simulink model "TestHarness"  (R2025b)
settings: Solver=VariableStepAuto  StartTime=0.0  StopTime=16  RelTol=1e-3  AbsTol=1e-3
PreLoadFcn:
  | SimulationTime = 10;
  | run('Harnessparm.m');
  | Choice=1;
undefined symbols (not defined in the file): base, Base, GFLBatteryController, loadl, pll, PVController, PVInverter, scan, Ts
libraries: nesl_utility x11, ee_lib x10, eeTransforms x7, fl_lib x5, eeSinusoidalMeasurementV2 x2, slpidlib x2, eeGeneralControl x2
settings Model: SimulationMode=accelerator  Creator=rajarshd  LastModifiedBy=rajarshd
settings SolverCC: AutoScaleAbsTol=off  AlgebraicLoopSolver=TrustRegion  MaxZcPerStep=1.0
settings DataIOCC: SaveOutput=off  DSMLogging=off  SaveTime=off  ReturnWorkspaceOutputsName=Data
settings DebuggingCC: UnconnectedInputMsg=warning  UnconnectedOutputMsg=warning  UnconnectedLineMsg=warning  SymbolicDimsDataTypeCodeGenerationDiagnostic=none
settings ModelReferenceCC: EnableRefExpFcnMdlSchedulingChecks=on
settings SFSimCC: CustomCodeUndefinedFunction=UseInterfaceOnly
settings RTWCC: GPUComputeCapability=3.5  DLArmComputeVersion=19.05
settings SimscapeCC: SimscapeLogType=all  SimscapeLogSimulationStatistics=on  SimscapeLogDataHistory=10000.0

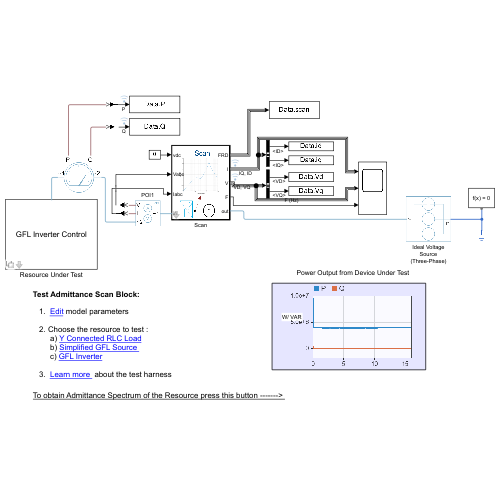
[thumbnail: Simulink's stored preview of the top-level diagram]
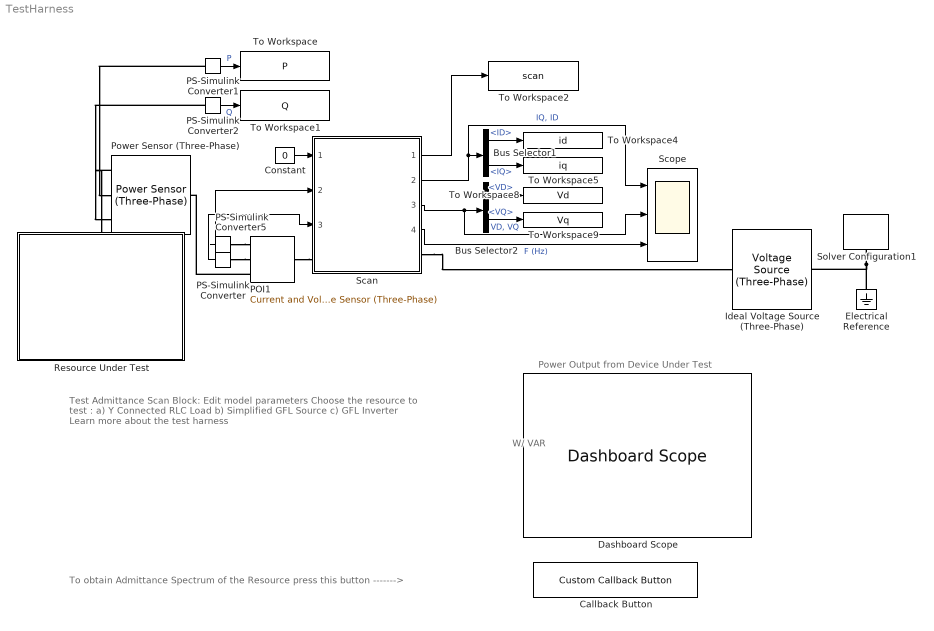
== system TestHarness ==
  note: W/ VAR
  note: Power Output from Device Under Test
  note: To obtain Admittance Spectrum of the Resource press this button ------->
  note: Test Admittance Scan Block:
      |
      | Edit model parameters
      |
      | Choose the resource to test :
      | a) Y Connected RLC Load
      | b) Simplified GFL Source
      | c) GFL Inverter
      |
      | Learn more about the test harness
  Bus Selector1 : BusSelector  OutputSignals=ID,IQ
  Bus Selector2 : BusSelector  OutputSignals=VD,VQ
  Callback Button : CustomCallbackButton  Configuration="{\"components\":[{\"name\":\"BackgroundImageComponent\",\"settings\":{\"image\":{\"size\":[0,0],\"src\":\"default\",\"srcOrientation\":\"Right\"},\"position\":[0,0,1,1]}},{\"name\":\"ButtonStateComponent\",\"settings\":{\"buttonType\":\"latch\",\"clickFcn\":\"Data=sim(bdroot);\\nmdl='TestHarness'; % Test model with IBR plant\\nadmittancescanPRBS(scan.Vd,scan.Vq,scan.Vdc,scan.f,Data.scan,modelorder,\\\"Y\\\") \",\"latched\":false,\"offValue\":null,\"onValue\":1,\"position\":[0,0,1,1],\"pressDelay\":\"500\",\"pressFcn\":\"\",\"repeatInterval\":\"0\",\"states\":[{\"horizontalAlignment\":\"center\",\"image\":{\"position\":[0,0,1,1],\"size\":[1,1],\"src\":\"default\",\"srcOrientation\":\"Right\"},\"label\":{\"color\":[1,1,1],\"icon\":{\"size\":[0,0],\"src\":\"default\",\"srcOrientation\":\"Right\"},\"iconOffset\":0,\"iconPlacement\":\"left\",\"opacity\":1,\"show\":true,\"text\":{\"content\":\"Admittance Scan\",\"font\":\"Helvetica\"}},\"labelOffset\":[0,0],\"verticalAlignment\":\"middle\"},{\"horizontalAlignment\":\"center\",\"image\":{\"position\":[0,0,1,1],\"size\":[1,1],\"src\":\"default\",\"srcOrientation\":\"Right\"},\"label\":{\"color\":[0.8509803921568627,0.3254901960784314,0.09803921568627451],\"icon\":{\"size\":[0,0],\"src\":\"default\",\"srcOrientation\":\"Right\"},\"iconOffset\":0,\"iconPlacement\":\"left\",\"opacity\":0,\"show\":true,\"text\":{\"content\":\"Admittance Scan\",\"font\":\"Helvetica\"}},\"labelOffset\":[-0.01428571428571429,-5.551115123125783e-17],\"verticalAlignment\":\"middle\"},{\"horizontalAlignment\":\"center\",\"image\":{\"position\":[0,0,1,1],\"size\":[1,1],\"src\":\"default\",\"srcOrientation\":\"Right\"},\"label\":{\"color\":[0.01176470588,0.01176470588,0.01176470588,1],\"icon\":{\"size\":[0,0],\"src\":\"default\",\"srcOrientation\":\"Right\"},\"iconOffset\":0,\"iconPlacement\":\"left\",\"opacity\":1,\"show\":true,\"text\":{\"content\":\"Admittance Scan\",\"font\":\"Helvetica\"}},\"labelOffset\":[0,0],\"verticalAlignment\":\"middle\"},{\"horizontalAlignment\":\"center\",\"image\":{\"position\":[0,0,1,1],\"size\":[1,1],\"src\":\"default\",\"srcOrientation\":\"Right\"},\"label\":{\"color\":[0.01176470588,0.01176470588,0.01176470588,1],\"icon\":{\"size\":[0,0],\"src\":\"default\",\"srcOrientation\":\"Right\"},\"iconOffset\":0,\"iconPlacement\":\"left\",\"opacity\":1,\"show\":true,\"text\":{\"content\":\"Admittance Scan\",\"font\":\"Helvetica\"}},\"labelOffset\":[0,0],\"verticalAlignment\":\"middle\"}]}},{\"name\":\"ForegroundImageComponent\",\"settings\":{\"image\":{\"size\":[0,0],\"src\":\"default\",\"srcOrientation\":\"Right\"},\"isForeground\":1,\"position\":[0,0,1,1]}}],\"derived\":{\"blockParameters\":{\"AutoActivate\":true,\"ButtonText\":\"Admittance Scan\",\"ButtonType\":\"Latch\",\"ClickFcn\":\"Data=sim(bdroot);\\nmdl='TestHarness'; % Test model with IBR plant\\nadmittancescanPRBS(scan.Vd,scan.Vq,scan.Vdc,scan.f,Data.scan,modelorder,\\\"Y\\\") \",\"OnValue\":1,\"PressDelay\":\"500\",\"PressFcn\":\"\",\"RepeatInterval\":\"0\",\"fixedAspectRatio\":\"off\"}},\"settings\":{\"BindingType\":\"standalone\",\"autoActivate\":true,\"backgroundColor\":[244,244,244,1],\"backgroundOffset\":0.2,\"backgroundOpacity\":1,\"fixedAspectRatio\":\"off\",\"foregroundColor\":[0.01176470588,0.01176470588,0.01176470588,1],\"migratedFromLegacy\":true,\"useBackgroundColor\":true,\"variant\":\"callback\",\"version\":\"R2025a\"},\"type\":\"Button\"}"  CustomBackgroundColor="{\"color\":[0,0.4470588235294118,0.7411764705882353],\"show\":true}"
  Constant : Constant  Value=0
  Dashboard Scope : DashboardScope  Ymin=0  Ymax=1e7  FontColor=[0.0, 0.0, 0.0]
  Electrical Reference : fl_lib/Electrical/Electrical Elements/Electrical Reference
  Ideal Voltage Source (Three-Phase) : ee_lib/Sources/Voltage Source (Three-Phase)  vline_rms=grid.voltage V  shift=0 deg  freq=grid.frequency Hz  impedance_option=0  SShortCircuit=1e6 A*V  XR=15  R=0.01 Ohm  L=0.2 mH  harmonic_option=0  harmonic_orders=[5, 7, 11, 13]  harmonic_ratios=[.1, .1, .1, .1]  G_parasitic=0 1/Ohm  I_specify=off  I_priority=None  I=[0, 0, 0] A  I_nominal_specify=off  I_nominal_value=1  I_nominal_unit=A
  POI1 : ee_lib/Sensors & Transducers/Current and Voltage Sensor (Three-Phase)  vMeasurementType=ee.enum.vmeasurement.lg  outputUnit=ee.enum.unit.si  SRated=base.mVA A*V  VRated=base.kV V  I_specify=off  I_priority=None  I=[0, 0, 0] A  I_nominal_specify=off  I_nominal_value=1  I_nominal_unit=A  V_specify=off  V_priority=None  V=[0, 0, 0] V  V_nominal_specify=off  V_nominal_value=1  V_nominal_unit=V
      settings: InternalSimscapePortConfiguration="{\"Bottom\":[],\"Left\":[{\"id\":\"N1\",\"label\":\"~1\",\"type\":\"foundation.electrical.three_phase\"}],\"Right\":[{\"id\":\"V_output\",\"label\":\"V\",\"type\":\"output\"},{\"id\":\"I_output\",\"label\":\"I\",\"type\":\"output\"},{\"id\":\"N2\",\"label\":\"~2\",\"type\":\"foundation.electrical.three_phase\"}],\"Top\":[]}"
  PS-Simulink Converter{,1..2,5} (4 alike) : nesl_utility/PS-Simulink Converter  PhysicalDomain=network_engine_domain  SubClassName=ps_output  LeftPortType=input  RightPortType=output  PseudoPeriodic=off  Frequencies=[]  VectorFormat=inherit  Unit=inherit  AffineConversion=off
  Power Sensor (Three-Phase) : ee_lib/Sensors & Transducers/Power Sensor (Three-Phase)  load_type=ee.enum.passive.type_balanced.balanced  f0=60 Hz
      settings: InternalSimscapePortConfiguration="{\"Bottom\":[],\"Left\":[{\"id\":\"N1\",\"label\":\"~1\",\"type\":\"foundation.electrical.three_phase\"}],\"Right\":[{\"id\":\"N2\",\"label\":\"~2\",\"type\":\"foundation.electrical.three_phase\"}],\"Top\":[{\"id\":\"Pm\",\"label\":\"P\",\"type\":\"output\"},{\"id\":\"Qm\",\"label\":\"Q\",\"type\":\"output\"}]}"
  Resource Under Test : Subsystem  Variant=on  VariantControl=Subsystem2  mask{Choice=GFL BESS}
      mask prompts: Choice "Choose Resource"
      mask TypeOptions Choice: Y Connected Load | Simplified GFL Source | GFL BESS
  Scan : Subsystem  ReferencedSubsystem=ScanBlockwithDC  F0=grid.frequency  Theta0=0  Kp_LF=pll.kp  Ki_LF=pll.ki  Ts=Ts  voltage=Base.KV_base_new  voltagedc=0  mva=base.mVA  Amplitude=scan.Vd  Amplitude1=scan.Vq  Amplitudedc=scan.Vdc  f=scan.f  T=1/scan.samplingfrequency  Tdis=scan.start  Tend=scan.end  VSelect=Equivalent Series Voltage (V)  Hold=No
  Scope : Scope  NumInputPorts=3
      settings: ActiveDisplayYMinimum=-3286.03322  ActiveDisplayYMaximum=550.92742
  Solver Configuration1 : nesl_utility/Solver Configuration  PhysicalDomain=network_engine_domain  SubClassName=solver  LeftPortType=input  RightPortType=generic  Tones=[]  Harmonics=[]  SimulateNoise=off  Profile=off  UseLocalSampling=off  EnableSwitchedLinearOptims=on  FrequencyDomain=off  UseCCode=off  RelTol=0.001  AbsTol=1e-06  MinStep=1e-09  ToWorkspace=off  RevertToSquareIcSolve=off  NumHomotopyIterations=100  PhasorMode=off  PhasorModeNumHarmonics=1  ConsistencySolver=NEWTON_XTOL_AFTER_FTOL  IndexReductionMethod=None  DoDC=off  ResidualTolerance=1e-3  ConsistencyTolSource=GLOBAL  ConsistencyAbsTol=0.001  ConsistencyRelTol=0.001  ConsistencyTolFactor=0.001  UseLocalSolver=on  LocalSolverChoice=NE_BACKWARD_EULER_ADVANCER  ResolveIndetEquations=off  FunctionEvalNumThread=1  LocalSolverSampleTime=5e-5  DoFixedCost=on  MaxNonlinIter=1  MaxModeIter=2  ComputeImpulses=off  ImpulseIterations=2  LinearAlgebra=Sparse  LinearAlgebraNumThread=0  EquationFormulation=NE_TIME_EF  DelaysMemoryBudget=1024  AutomaticFiltering=on  FilteringTimeConstant=0.001  PartitionStorageMethod=AS_NEEDED  PartitionMemoryBudget=1024  PartitionMethod=ROBUST  MultibodyUseLocalSolver=off  MultibodyLocalSolverChoice=ODE1  MultibodyLocalSolverSampleTime=0.001
  To Workspace : ToWorkspace  VariableName=P  SaveFormat=Timeseries  SampleTime=-1
  To Workspace1 : ToWorkspace  VariableName=Q  SaveFormat=Timeseries  SampleTime=-1
  To Workspace2 : ToWorkspace  VariableName=scan  SaveFormat=Timeseries  SampleTime=-1
  To Workspace4 : ToWorkspace  VariableName=id  SaveFormat=Timeseries  SampleTime=-1
  To Workspace5 : ToWorkspace  VariableName=iq  SaveFormat=Timeseries  SampleTime=-1
  To Workspace8 : ToWorkspace  VariableName=Vd  SaveFormat=Timeseries  SampleTime=-1
  To Workspace9 : ToWorkspace  VariableName=Vq  SaveFormat=Timeseries  SampleTime=-1
  wires:
  PS-Simulink Converter1/1 -> To Workspace/1  "P"
  PS-Simulink Converter2/1 -> To Workspace1/1  "Q"
  Scan/2 -> Scope/1, Bus Selector1/1  "IQ, ID"
  Scan/1 -> To Workspace2/1
  Scan/4 -> Scope/3  "F (Hz)"
  Scan/3 -> Scope/2, Bus Selector2/1  "VD, VQ"
  Bus Selector1/1 -> To Workspace4/1  "<ID>"
  Bus Selector1/2 -> To Workspace5/1  "<IQ>"
  Bus Selector2/1 -> To Workspace8/1  "<VD>"
  Bus Selector2/2 -> To Workspace9/1  "<VQ>"
  Constant/1 -> Scan/1
  PS-Simulink Converter5/1 -> Scan/2
  PS-Simulink Converter/1 -> Scan/3
  connections:
  PS-Simulink Converter1/LConn1 -- Power Sensor (Three-Phase)/LConn2
  PS-Simulink Converter2/LConn1 -- Power Sensor (Three-Phase)/LConn3
  Scan/RConn1 -- Ideal Voltage Source (Three-Phase)/RConn1
  Solver Configuration1/RConn1 -- Ideal Voltage Source (Three-Phase)/LConn1 -- Electrical Reference/LConn1
  PS-Simulink Converter/LConn1 -- POI1/RConn2
  PS-Simulink Converter5/LConn1 -- POI1/RConn1
  Power Sensor (Three-Phase)/LConn1 -- Resource Under Test/LConn1
  POI1/LConn1 -- Scan/LConn1
  POI1/RConn3 -- Power Sensor (Three-Phase)/RConn1

== system TestHarness/Resource Under Test ==
  " GFL Source" : Subsystem  VariantControl=Choice==2  mask{axis=D Axis, Denominator=[1 2*0.1*(2*pi*40) (2*pi*40)^2], Numerator=1e3, Numerator1=1e3, Denominator1=[1 +2*0.1*(2*pi*40) (2*pi*40)^2]}
      mask prompts: axis "TF Along:"; Denominator "D axis TF Denominator"; Numerator "D axis TF Numerator"; Numerator1 "Q axis TF Numerator"; Denominator1 "Q axis TF Denominator"
      mask TypeOptions axis: D Axis | Q Axis
      mask Display:
      | g=get_param(gcb,'axis');
      | if(g=='D Axis')
      | den = get_param(gcb, 'Denominator');
      | nu  = get_param(gcb, 'Numerator');
      | disp('Admittance TF along D axis:\n\n\n\n\n');
      | den1 = get_param(gcb, 'Denominator1');
      | nu1  = get_param(gcb, 'Numerator1');
      | dpoly(nu, den,'s');
      | end
      | if(g=='Q Axis')
      | den1 = get_param(gcb, 'Denominator1');
      | nu1  = get_param(gcb, 'Numerator1');
      | disp('Admittance TF along Q axis:\n\n\n\n\n');
      | den1 = get_param(gcb, 'Denominator1');
      | nu1  = get_param(gcb, 'Numerator1');
      | dpoly(nu1, den1,'s');
      | end
  GFL : Subsystem  VariantControl=Choice==3
      mask Display: disp('GFL Inverter Control');
  Wye-Connected Load : Subsystem  VariantControl=Choice==1  mask{C=loadl.c, L=loadl.l, R=loadl.r}
      mask prompts: C "physmod:ee:library:comments:passive:rlc_assemblies:wye:Xabc:C"; L "physmod:ee:library:comments:passive:rlc_assemblies:wye:Xabc:L"; R "physmod:ee:library:comments:passive:rlc_assemblies:wye:Xabc:R"
      mask TypeOptions C: Wye-Connected Load/C
      mask TypeOptions L: Wye-Connected Load/L
      mask TypeOptions R: Wye-Connected Load/R
      mask Display: disp('Y Connected \n R L C series Load');
  Conn1 : PMIOPort  Side=Left

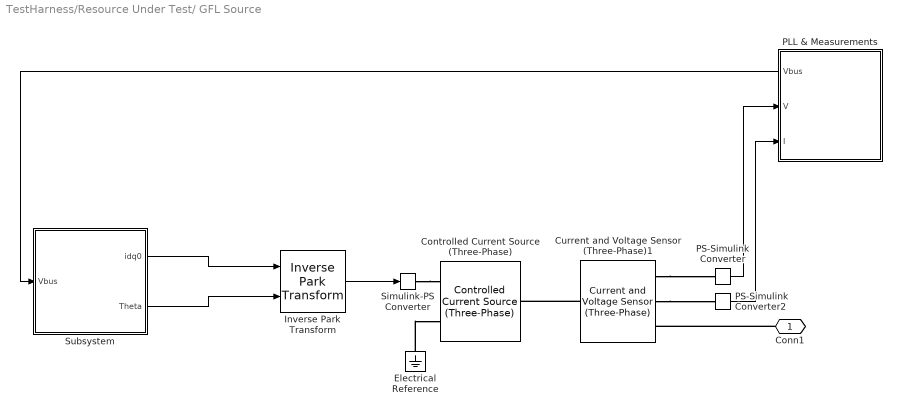
== system TestHarness/Resource Under Test/ GFL Source ==
  Controlled Current Source (Three-Phase) : ee_lib/Sources/Controlled Current Source (Three-Phase)  input_option=ee.enum.inputType.instantaneous  FRated=60 Hz
      settings: InternalSimscapePortConfiguration="{\"Bottom\":[],\"Left\":[{\"id\":\"S\",\"label\":\"S\",\"type\":\"input\"},{\"id\":\"n\",\"label\":\"n\",\"type\":\"foundation.electrical.electrical\"}],\"Right\":[{\"id\":\"N\",\"label\":\"~\",\"type\":\"foundation.electrical.three_phase\"}],\"Top\":[]}"
  Current and Voltage Sensor (Three-Phase)1 : ee_lib/Sensors & Transducers/Current and Voltage Sensor (Three-Phase)  vMeasurementType=ee.enum.vmeasurement.lg  outputUnit=ee.enum.unit.si  SRated=base.mVA A*V  VRated=base.kV V  I_specify=off  I_priority=None  I=[0, 0, 0] A  I_nominal_specify=off  I_nominal_value=1  I_nominal_unit=A  V_specify=off  V_priority=None  V=[0, 0, 0] V  V_nominal_specify=off  V_nominal_value=1  V_nominal_unit=V
      settings: InternalSimscapePortConfiguration="{\"Bottom\":[],\"Left\":[{\"id\":\"N1\",\"label\":\"~1\",\"type\":\"foundation.electrical.three_phase\"}],\"Right\":[{\"id\":\"V_output\",\"label\":\"V\",\"type\":\"output\"},{\"id\":\"I_output\",\"label\":\"I\",\"type\":\"output\"},{\"id\":\"N2\",\"label\":\"~2\",\"type\":\"foundation.electrical.three_phase\"}],\"Top\":[]}"
  Electrical Reference : fl_lib/Electrical/Electrical Elements/Electrical Reference
  Inverse Park Transform : eeTransforms/Inverse Park Transform  AxisAlignment=Q-axis  PowerInvariant=on
      settings: LibrarySourceBlock=|
      | ee_sl_lib/Mathematical
      | Transforms/Inverse
      | Park Transform
  PLL & Measurements : Subsystem
      settings: PortSchema="{\"entries\":[{\"content\":{\"sides\":[{\"content\":{\"connectorIds\":[\"Out1\",\"In1\",\"In2\"]},\"type\":\"ConnectorPlacement.EquallySpacedRectSide\",\"uuid\":\"76485780-20fe-4fcf-8224-69648da6ed2a\"},{\"content\":{\"connectorIds\":[],\"side\":\"RIGHT\"},\"type\":\"ConnectorPlacement.EquallySpacedRectSide\",\"uuid\":\"f19a6390-e634-42c7-8d46-4cd80cbab182\"},{\"content\":{\"connectorIds\":[],\"side\":\"TOP\"},\"type\":\"ConnectorPlacement.EquallySpacedRectSide\",\"uuid\":\"87682f72-1844-428e-be70-ad7ca3191ee3\"}]},\"type\":\"ConnectorPlacement.EquallySpacedConnector\",\"uuid\":\"f2136b07-48ec-402b-adb3-18c0bac2157c\"}],\"packageUris\":[\"http://schema.mathworks.com/mf0/Connector/R2020b\"],\"version\":\"1.0\"}"
      mask Display: image('$imagefile'); % Use "Edit Image" on toolstrip to change.
  PS-Simulink Converter : nesl_utility/PS-Simulink Converter  PhysicalDomain=network_engine_domain  SubClassName=ps_output  LeftPortType=input  RightPortType=output  PseudoPeriodic=off  Frequencies=[]  VectorFormat=inherit  Unit=inherit  AffineConversion=off
  PS-Simulink Converter2 : nesl_utility/PS-Simulink Converter  PhysicalDomain=network_engine_domain  SubClassName=ps_output  LeftPortType=input  RightPortType=output  PseudoPeriodic=off  Frequencies=[]  VectorFormat=inherit  Unit=inherit  AffineConversion=off
  Simulink-PS Converter : nesl_utility/Simulink-PS Converter  PhysicalDomain=network_engine_domain  SubClassName=ps_input  LeftPortType=input  RightPortType=output  PseudoPeriodic=off  Frequencies=[]  NoiseDistribution=none  NoiseParameters=[]  Unit=1  AffineConversion=off  FilteringAndDerivatives=provide  SimscapeFilterOrder=1  InputFilterTimeConstant=0.001  UdotUserProvided=0
  Subsystem : Subsystem
  Conn1 : PMIOPort  Side=Left
  wires:
  PS-Simulink Converter/1 -> PLL & Measurements/1(V)
  PS-Simulink Converter2/1 -> PLL & Measurements/2(I)
  PLL & Measurements/1(Vbus) -> Subsystem/1(Vbus)
  Subsystem/1(idq0) -> Inverse Park Transform/1
  Inverse Park Transform/1 -> Simulink-PS Converter/1
  Subsystem/2(Theta) -> Inverse Park Transform/2
  connections:
  Current and Voltage Sensor (Three-Phase)1/RConn2 -- PS-Simulink Converter2/LConn1
  Current and Voltage Sensor (Three-Phase)1/RConn1 -- PS-Simulink Converter/LConn1
  Simulink-PS Converter/RConn1 -- Controlled Current Source (Three-Phase)/LConn1
  Electrical Reference/LConn1 -- Controlled Current Source (Three-Phase)/LConn2
  Conn1/RConn1 -- Current and Voltage Sensor (Three-Phase)1/RConn3
  Current and Voltage Sensor (Three-Phase)1/LConn1 -- Controlled Current Source (Three-Phase)/RConn1

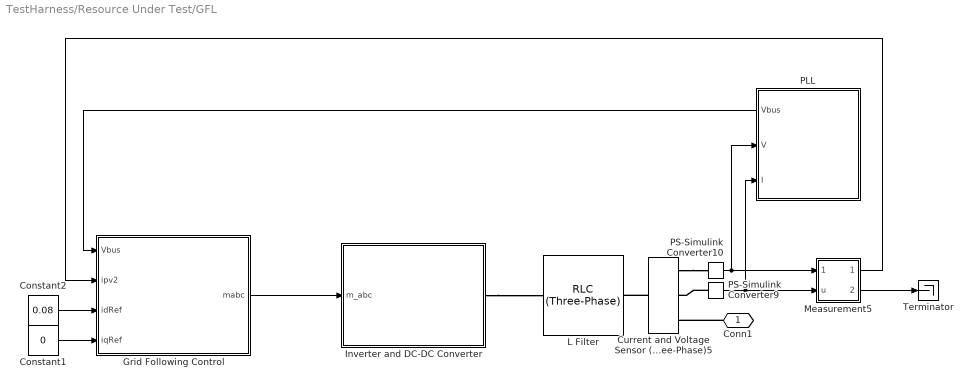
== system TestHarness/Resource Under Test/GFL ==
  Constant1 : Constant  Value=0  SampleTime=Ts
  Constant2 : Constant  Value=0.08  SampleTime=Ts
  Current and Voltage Sensor (Three-Phase)5 : ee_lib/Sensors & Transducers/Current and Voltage Sensor (Three-Phase)  vMeasurementType=ee.enum.vmeasurement.lg  outputUnit=ee.enum.unit.pu  SRated=Base.MVA_base_new A*V  VRated=Base.KV_base_new V  I_specify=off  I_priority=None  I=[0, 0, 0] A  I_nominal_specify=off  I_nominal_value=1  I_nominal_unit=A  V_specify=off  V_priority=None  V=[0, 0, 0] V  V_nominal_specify=off  V_nominal_value=1  V_nominal_unit=V
      settings: InternalSimscapePortConfiguration="{\"Bottom\":[],\"Left\":[{\"id\":\"N1\",\"label\":\"~1\",\"type\":\"foundation.electrical.three_phase\"}],\"Right\":[{\"id\":\"V_output\",\"label\":\"V\",\"type\":\"output\"},{\"id\":\"I_output\",\"label\":\"I\",\"type\":\"output\"},{\"id\":\"N2\",\"label\":\"~2\",\"type\":\"foundation.electrical.three_phase\"}],\"Top\":[]}"
  Grid Following Control : Subsystem  VariantControl=BESSGridSupporting
      mask Display: image('$imagefile'); % Use "Edit Image" on toolstrip to change.
  Inverter and DC-DC Converter : Subsystem
  L Filter : ee_lib/Passive/RLC Assemblies/RLC (Three-Phase)  port_option=ee.enum.threePhasePort.composite  component_structure=ee.enum.rlc.structure.L  R=1e-3 Ohm  L=PVInverter.L*10 H  C=1e-6 F  R_parasitic=0 Ohm  G_parasitic=0 1/Ohm  IL_specify=off  IL_priority=High  IL=[0, 0, 0] A  IL_nominal_specify=off  IL_nominal_value=1  IL_nominal_unit=A  VC_specify=off  VC_priority=High  VC=[0, 0, 0] V  VC_nominal_specify=off  VC_nominal_value=1  VC_nominal_unit=V
      settings: InternalSimscapePortConfiguration="{\"Bottom\":[],\"Left\":[{\"id\":\"N1\",\"label\":\"~1\",\"type\":\"foundation.electrical.three_phase\"}],\"Right\":[{\"id\":\"N2\",\"label\":\"~2\",\"type\":\"foundation.electrical.three_phase\"}],\"Top\":[]}"
  Measurement5 : Subsystem
  "PLL " : Subsystem
      settings: PortSchema="{\"entries\":[{\"content\":{\"sides\":[{\"content\":{\"connectorIds\":[\"Out1\",\"In1\",\"In2\"]},\"type\":\"ConnectorPlacement.EquallySpacedRectSide\",\"uuid\":\"76485780-20fe-4fcf-8224-69648da6ed2a\"},{\"content\":{\"connectorIds\":[],\"side\":\"RIGHT\"},\"type\":\"ConnectorPlacement.EquallySpacedRectSide\",\"uuid\":\"f19a6390-e634-42c7-8d46-4cd80cbab182\"},{\"content\":{\"connectorIds\":[],\"side\":\"TOP\"},\"type\":\"ConnectorPlacement.EquallySpacedRectSide\",\"uuid\":\"87682f72-1844-428e-be70-ad7ca3191ee3\"}]},\"type\":\"ConnectorPlacement.EquallySpacedConnector\",\"uuid\":\"f2136b07-48ec-402b-adb3-18c0bac2157c\"}],\"packageUris\":[\"http://schema.mathworks.com/mf0/Connector/R2020b\"],\"version\":\"1.0\"}"
      mask Display: image('$imagefile'); % Use "Edit Image" on toolstrip to change.
  PS-Simulink Converter10 : nesl_utility/PS-Simulink Converter  PhysicalDomain=network_engine_domain  SubClassName=ps_output  LeftPortType=input  RightPortType=output  PseudoPeriodic=off  Frequencies=[]  VectorFormat=inherit  Unit=inherit  AffineConversion=off
  PS-Simulink Converter9 : nesl_utility/PS-Simulink Converter  PhysicalDomain=network_engine_domain  SubClassName=ps_output  LeftPortType=input  RightPortType=output  PseudoPeriodic=off  Frequencies=[]  VectorFormat=inherit  Unit=inherit  AffineConversion=off
  Terminator : Terminator
  Conn1 : PMIOPort  Side=Left
  wires:
  Grid Following Control/1(mabc) -> Inverter and DC-DC Converter/1(m_abc)
  PS-Simulink Converter9/1 -> "PLL "/2(I), Measurement5/2(u)
  PS-Simulink Converter10/1 -> "PLL "/1(V), Measurement5/1(In1)
  Measurement5/2(Bat) -> Terminator/1
  Measurement5/1(ipv1) -> Grid Following Control/2(ipv2)
  "PLL "/1(Vbus) -> Grid Following Control/1(Vbus)
  Constant2/1 -> Grid Following Control/3(idRef)
  Constant1/1 -> Grid Following Control/4(iqRef)
  connections:
  Conn1/RConn1 -- Current and Voltage Sensor (Three-Phase)5/RConn3
  Inverter and DC-DC Converter/RConn1 -- L Filter/LConn1
  Current and Voltage Sensor (Three-Phase)5/LConn1 -- L Filter/RConn1
  Current and Voltage Sensor (Three-Phase)5/RConn1 -- PS-Simulink Converter10/LConn1
  PS-Simulink Converter9/LConn1 -- Current and Voltage Sensor (Three-Phase)5/RConn2

== system TestHarness/Resource Under Test/Wye-Connected Load ==
  Electrical Reference : fl_lib/Electrical/Electrical Elements/Electrical Reference
  Wye-Connected Load : ee_lib/Passive/RLC Assemblies/Wye-Connected Load  port_option=ee.enum.threePhasePort.composite  parameterization=ee.enum.rlc.parameterization.direct  component_structure=ee.enum.rlc.structure.SeriesRLC  component_structure_PQ=ee.enum.rlc.structure.SeriesRL  R=R Ohm  L=L H  C=C F  VRated=24e3 V  FRated=60 Hz  P=1e3 W  Qpos=1e2 A*V  Qneg=-1e2 A*V  R_parasitic=0 Ohm  G_parasitic=0 1/Ohm  R_parasitic_PQ=0 Ohm  G_parasitic_PQ=0 1/Ohm  Vmag0=24e3 V  Vang0=0 deg  Freq0=60 Hz  IL_specify=off  IL_priority=High  IL=[0, 0, 0] A  IL_nominal_specify=off  IL_nominal_value=1  IL_nominal_unit=A  VC_specify=off  VC_priority=High  VC=[0, 0, 0] V  VC_nominal_specify=off  VC_nominal_value=1  VC_nominal_unit=V
  Conn1 : PMIOPort  Side=Left
  connections:
  Conn1/RConn1 -- Wye-Connected Load/LConn1
  Electrical Reference/LConn1 -- Wye-Connected Load/RConn1

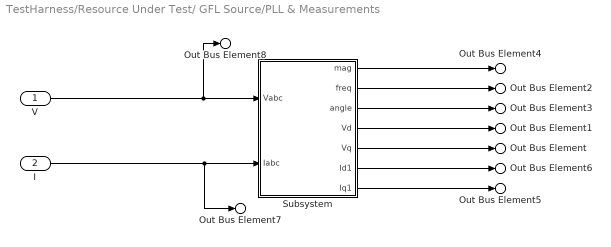
== system TestHarness/Resource Under Test/ GFL Source/PLL & Measurements ==
  V : Inport
  I : Inport  Port=2
  Subsystem : Subsystem
  Out Bus Element : Outport  PortName=Vbus  Element=Vq
  Out Bus Element1 : Outport  PortName=Vbus  Element=Vd
  Out Bus Element2 : Outport  PortName=Vbus  Element=w
  Out Bus Element3 : Outport  PortName=Vbus  Element=Theta
  Out Bus Element4 : Outport  PortName=Vbus  Element=Vmag
  Out Bus Element5 : Outport  PortName=Vbus  Element=Iq
  Out Bus Element6 : Outport  PortName=Vbus  Element=Id
  Out Bus Element7 : Outport  PortName=Vbus  Element=Iabc
  Out Bus Element8 : Outport  PortName=Vbus  Element=Vabc
  wires:
  Subsystem/2(freq) -> Out Bus Element2/1
  Subsystem/5(Vq) -> Out Bus Element/1
  Subsystem/3(angle) -> Out Bus Element3/1
  Subsystem/4(Vd) -> Out Bus Element1/1
  V/1 -> Out Bus Element8/1, Subsystem/1(Vabc)
  Subsystem/1(mag) -> Out Bus Element4/1
  I/1 -> Out Bus Element7/1, Subsystem/2(Iabc)
  Subsystem/7(Iq1) -> Out Bus Element5/1
  Subsystem/6(Id1) -> Out Bus Element6/1

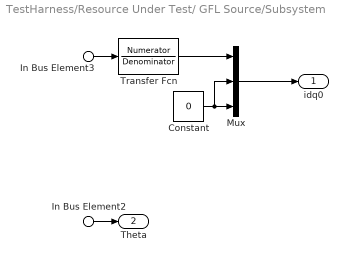
== system TestHarness/Resource Under Test/ GFL Source/Subsystem ==
  In Bus Element3 : Inport  PortName=Vbus  Element=Vd
  In Bus Element2 : Inport  PortName=Vbus  Element=Theta
  Constant : Constant  Value=0
  Mux : Mux  Inputs=3
  Transfer Fcn : TransferFcn  Numerator=Numerator  Denominator=Denominator
  idq0 : Outport
  Theta : Outport  Port=2
  wires:
  Mux/1 -> idq0/1
  In Bus Element2/1 -> Theta/1
  In Bus Element3/1 -> Transfer Fcn/1
  Constant/1 -> Mux/2, Mux/3
  Transfer Fcn/1 -> Mux/1

== system TestHarness/Resource Under Test/GFL/Grid Following Control ==
  In Bus Element : Inport  PortName=Vbus
  In Bus Element1 : Inport  Port=2  PortName=ipv2
  idRef : Inport  Port=3
  iqRef : Inport  Port=4
  GFL Battery Controller : Subsystem  mask{Vref=GFLBatteryController.V_ref, fref=GFLBatteryController.f_ref, Pref=GFLBatteryController.P_ref, Qref=GFLBatteryController.Q_ref, mp=GFLBatteryController.m_p, mv=GFLBatteryController.m_v, P=Real power, MVA=Base.MVA_base_new, zbase=Base.z_base, L=PVInverter.L*10, Imax=PVInverter.I_max_pu, Td=GFLBatteryController.Td, Kpic=PVController.Kp_ic, Kiic=PVController.Ki_ic, Kd=PVController.Kd}
      mask prompts: Vref "Voltage reference (PU)"; fref "Frequency reference (Hz)"; Pref "Real power reference (PU)"; Qref "Reactive power reference (PU)"; mp "Real power droop cofficient"; mv "Reactive power droop cofficient"; P "Priority mode"; MVA "Base Power (V*A)"; zbase "Base Impedance (Ohm)"; L "Filter Inductance (H)"; Imax "Inverter current limit (pu)"; Td "Sensor time delay (s)"; Kpic "Proportional gain"; Kiic "Integral gain"; Kd "Derevative gain"
      mask TypeOptions P: Real power  | Reactive power
      mask DialogControl Container4 Prompt: General
      mask DialogControl Container5 Prompt: Current Controller
      mask Display: image('$imagefile'); % Use "Edit Image" on toolstrip to change.
  mabc : Outport
  wires:
  In Bus Element/1 -> GFL Battery Controller/1(Vbus)
  In Bus Element1/1 -> GFL Battery Controller/2(ipv2)
  GFL Battery Controller/1(m_abc) -> mabc/1
  idRef/1 -> GFL Battery Controller/3(IdRef)
  iqRef/1 -> GFL Battery Controller/4(IqRef)

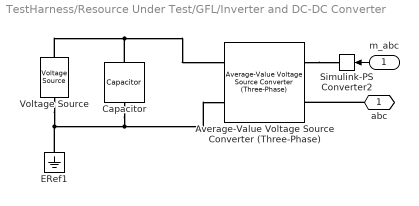
== system TestHarness/Resource Under Test/GFL/Inverter and DC-DC Converter ==
  m_abc : Inport
  Average-Value Voltage Source Converter (Three-Phase) : ee_lib/Semiconductors & Converters/Converters/Average-Value Voltage Source Converter (Three-Phase)  port_option=ee.enum.threePhasePort.composite  frequency_option=ee.enum.converters.frequency.variable  input_option=ee.enum.converters.inputOption.ModWave  FRated=60 Hz  losses_parameterization=ee.enum.converters.losses.fixed  Pfixed=1 W  ks=0.01  kc1=1.7 V  kc2=0.01 Ohm  Ploss_vect=[100, 800, 1870, 3250, 4900] W  Irms_vect=[10, 100, 200, 300, 400] A  Vdc_nom=300 V  thermal_mass=30000 J/K  temperature_specify=off  temperature_priority=High  temperature=298.15 K  temperature_nominal_specify=off  temperature_nominal_value=1  temperature_nominal_unit=K
      settings: InternalSimscapePortConfiguration="{\"Bottom\":[],\"Left\":[{\"id\":\"ModWave\",\"label\":\"ModWave\",\"type\":\"input\"},{\"id\":\"N\",\"label\":\"~\",\"type\":\"foundation.electrical.three_phase\"}],\"Right\":[{\"id\":\"p\",\"label\":\"+\",\"type\":\"foundation.electrical.electrical\"},{\"id\":\"n\",\"label\":\"-\",\"type\":\"foundation.electrical.electrical\"}],\"Top\":[]}"
  Capacitor : fl_lib/Electrical/Electrical Elements/Capacitor  c=GFMBatteryController.C_dc F  r=1e-6 Ohm  g=0 1/Ohm  i_specify=off  i_priority=None  i=0 A  i_nominal_specify=off  i_nominal_value=1  i_nominal_unit=A  v_specify=off  v_priority=None  v=6560*.5 V  v_nominal_specify=off  v_nominal_value=1  v_nominal_unit=V  vc_specify=on  vc_priority=None  vc=PVInverter.Vdc V  vc_nominal_specify=off  vc_nominal_value=1  vc_nominal_unit=V
  ERef1 : fl_lib/Electrical/Electrical Elements/Electrical Reference
  Simulink-PS Converter2 : nesl_utility/Simulink-PS Converter  PhysicalDomain=network_engine_domain  SubClassName=ps_input  LeftPortType=input  RightPortType=output  PseudoPeriodic=off  Frequencies=[]  NoiseDistribution=none  NoiseParameters=[]  Unit=1  AffineConversion=off  FilteringAndDerivatives=provide  SimscapeFilterOrder=1  InputFilterTimeConstant=0.001  UdotUserProvided=0
  Voltage Source : ee_lib/Sources/Voltage Source  dc_voltage=PVInverter.Vdc V  ac_voltage=0 V  ac_shift=0 rad  ac_frequency=60 Hz  noise_mode=ee.enum.sources.noise.Disabled  PSD=0 V^2/Hz  sample_time=1e-3 s  repeatability=ee.enum.sources.repeatability.NotRepeatable  user_seed=0  auto_seed=1872246315  i_specify=off  i_priority=None  i=0 A  i_nominal_specify=off  i_nominal_value=1  i_nominal_unit=A  v_specify=off  v_priority=None  v=0 V  v_nominal_specify=off  v_nominal_value=1  v_nominal_unit=V
  abc : PMIOPort  Side=Right
  wires:
  m_abc/1 -> Simulink-PS Converter2/1
  connections:
  Voltage Source/RConn1 -- ERef1/LConn1 -- Capacitor/RConn1 -- Average-Value Voltage Source Converter (Three-Phase)/RConn2
  Capacitor/LConn1 -- Voltage Source/LConn1 -- Average-Value Voltage Source Converter (Three-Phase)/RConn1
  Average-Value Voltage Source Converter (Three-Phase)/LConn1 -- Simulink-PS Converter2/RConn1
  abc/RConn1 -- Average-Value Voltage Source Converter (Three-Phase)/LConn2

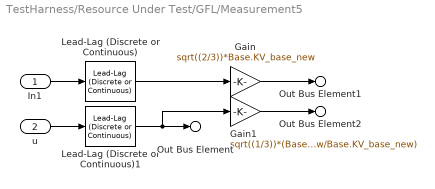
== system TestHarness/Resource Under Test/GFL/Measurement5 ==
  In1 : Inport
  u : Inport  Port=2
  Gain : Gain  Gain=sqrt((2/3))*Base.KV_base_new
  Gain1 : Gain  Gain=sqrt((1/3))*(Base.MVA_base_new/Base.KV_base_new)
  Lead-Lag (Discrete or Continuous) : eeGeneralControl/Lead-Lag (Discrete or Continuous)  T1=0  T2=PVController.t_sensor  B=inf  A=-inf  init_option=Inherited from block input  x0=0  Ts=Ts
      settings: LibrarySourceBlock=|
      | ee_sl_lib/General Control/Lead-Lag
      | (Discrete or Continuous)
  Lead-Lag (Discrete or Continuous)1 : eeGeneralControl/Lead-Lag (Discrete or Continuous)  T1=0  T2=PVController.t_sensor  B=inf  A=-inf  init_option=Inherited from block input  x0=0  Ts=Ts
      settings: LibrarySourceBlock=|
      | ee_sl_lib/General Control/Lead-Lag
      | (Discrete or Continuous)
  Out Bus Element : Outport  PortName=ipv1  Element=1
  Out Bus Element1 : Outport  Port=2  PortName=Bat  Element=Vabc_bat
  Out Bus Element2 : Outport  Port=2  PortName=Bat  Element=Iabc_bat
  wires:
  u/1 -> Lead-Lag (Discrete or Continuous)1/1
  Lead-Lag (Discrete or Continuous)1/1 -> Gain1/1, Out Bus Element/1
  In1/1 -> Lead-Lag (Discrete or Continuous)/1
  Lead-Lag (Discrete or Continuous)/1 -> Gain/1
  Gain/1 -> Out Bus Element1/1
  Gain1/1 -> Out Bus Element2/1

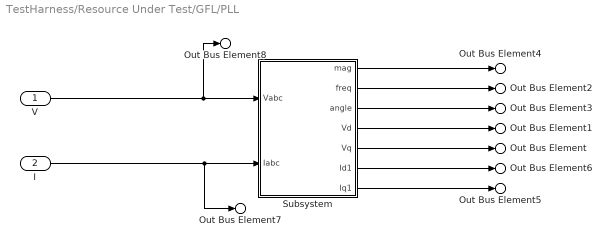
== system TestHarness/Resource Under Test/GFL/PLL  ==
  V : Inport
  I : Inport  Port=2
  Subsystem : Subsystem
  Out Bus Element : Outport  PortName=Vbus  Element=Vq
  Out Bus Element1 : Outport  PortName=Vbus  Element=Vd
  Out Bus Element2 : Outport  PortName=Vbus  Element=w
  Out Bus Element3 : Outport  PortName=Vbus  Element=Theta
  Out Bus Element4 : Outport  PortName=Vbus  Element=Vmag
  Out Bus Element5 : Outport  PortName=Vbus  Element=Iq
  Out Bus Element6 : Outport  PortName=Vbus  Element=Id
  Out Bus Element7 : Outport  PortName=Vbus  Element=Iabc
  Out Bus Element8 : Outport  PortName=Vbus  Element=Vabc
  wires:
  Subsystem/2(freq) -> Out Bus Element2/1
  Subsystem/5(Vq) -> Out Bus Element/1
  Subsystem/3(angle) -> Out Bus Element3/1
  Subsystem/4(Vd) -> Out Bus Element1/1
  V/1 -> Out Bus Element8/1, Subsystem/1(Vabc)
  Subsystem/1(mag) -> Out Bus Element4/1
  I/1 -> Out Bus Element7/1, Subsystem/2(Iabc)
  Subsystem/7(Iq1) -> Out Bus Element5/1
  Subsystem/6(Id1) -> Out Bus Element6/1

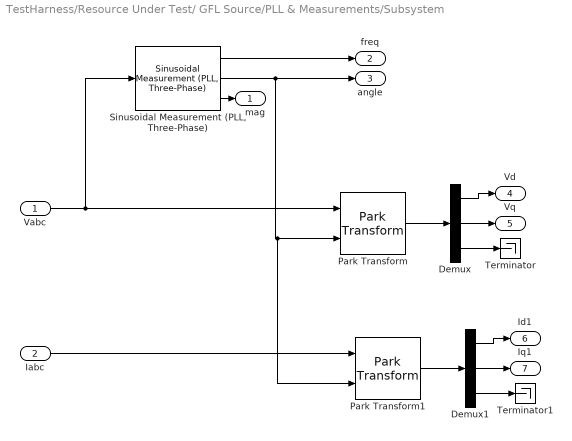
== system TestHarness/Resource Under Test/ GFL Source/PLL & Measurements/Subsystem ==
  Vabc : Inport
  Iabc : Inport  Port=2
  Demux : Demux  Outputs=3
  Demux1 : Demux  Outputs=3
  Park Transform : eeTransforms/Park Transform  AxisAlignment=Q-axis  PowerInvariant=on
  Park Transform1 : eeTransforms/Park Transform  AxisAlignment=Q-axis  PowerInvariant=on
  "Sinusoidal Measurement (PLL, Three-Phase)" : eeSinusoidalMeasurementV2/Sinusoidal Measurement (PLL, Three-Phase)  InputFilter=on  InputNormalization=off  Kp_LF=pll.kp/base.kV  Ki_LF=pll.ki /base.kV  F0=grid.frequency  Theta0=0  Ts=Ts
  Terminator : Terminator
  Terminator1 : Terminator
  mag : Outport
  freq : Outport  Port=2
  angle : Outport  Port=3
  Vd : Outport  Port=4
  Vq : Outport  Port=5
  Id1 : Outport  Port=6
  Iq1 : Outport  Port=7
  wires:
  Demux/3 -> Terminator/1
  Park Transform/1 -> Demux/1
  Demux/1 -> Vd/1
  Demux/2 -> Vq/1
  "Sinusoidal Measurement (PLL, Three-Phase)"/2 -> angle/1, Park Transform1/2, Park Transform/2
  "Sinusoidal Measurement (PLL, Three-Phase)"/1 -> freq/1
  "Sinusoidal Measurement (PLL, Three-Phase)"/3 -> mag/1
  Park Transform1/1 -> Demux1/1
  Demux1/1 -> Id1/1
  Demux1/2 -> Iq1/1
  Demux1/3 -> Terminator1/1
  Iabc/1 -> Park Transform1/1
  Vabc/1 -> "Sinusoidal Measurement (PLL, Three-Phase)"/1, Park Transform/1

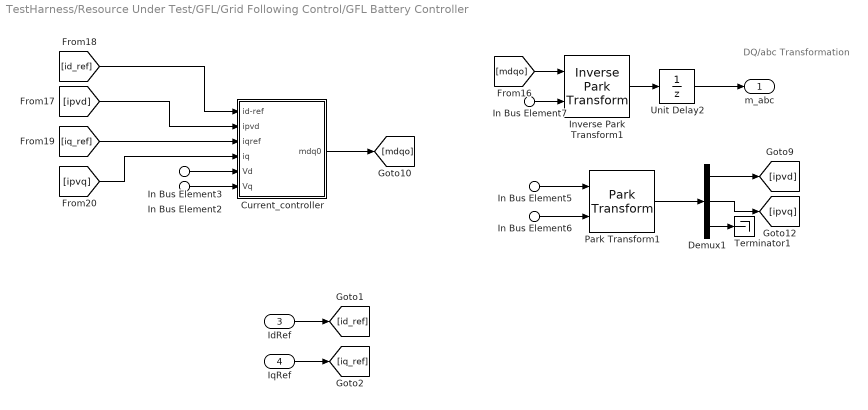
== system TestHarness/Resource Under Test/GFL/Grid Following Control/GFL Battery Controller ==
  note: DQ/abc Transformation
  In Bus Element3 : Inport  PortName=Vbus  Element=Vd
  In Bus Element2 : Inport  PortName=Vbus  Element=Vq
  In Bus Element6 : Inport  PortName=Vbus  Element=Theta
  In Bus Element7 : Inport  PortName=Vbus  Element=Theta
  In Bus Element5 : Inport  Port=2  PortName=ipv2  Element=1
  IdRef : Inport  Port=3
  IqRef : Inport  Port=4
  Current_controller : Subsystem
  Demux1 : Demux  Outputs=3
  Inverse Park Transform1 : eeTransforms/Inverse Park Transform  AxisAlignment=Q-axis  PowerInvariant=off
  Park Transform1 : eeTransforms/Park Transform  AxisAlignment=Q-axis  PowerInvariant=off
  Terminator1 : Terminator
  Unit Delay2 : UnitDelay  SampleTime=Ts  HasFrameUpgradeWarning=on
  m_abc : Outport
  wires:
  In Bus Element2/1 -> Current_controller/6(Vq)
  Current_controller/1(mdq0) -> [mdqo]
  Inverse Park Transform1/1 -> Unit Delay2/1
  Demux1/2 -> [ipvq]
  Unit Delay2/1 -> m_abc/1
  Demux1/1 -> [ipvd]
  Demux1/3 -> Terminator1/1
  [mdqo] -> Inverse Park Transform1/1
  Park Transform1/1 -> Demux1/1
  [id_ref] -> Current_controller/1(id-ref)
  In Bus Element3/1 -> Current_controller/5(Vd)
  [iq_ref] -> Current_controller/3(iqref)
  [ipvq] -> Current_controller/4(iq)
  In Bus Element6/1 -> Park Transform1/2
  In Bus Element7/1 -> Inverse Park Transform1/2
  [ipvd] -> Current_controller/2(ipvd)
  In Bus Element5/1 -> Park Transform1/1
  IqRef/1 -> [iq_ref]
  IdRef/1 -> [id_ref]

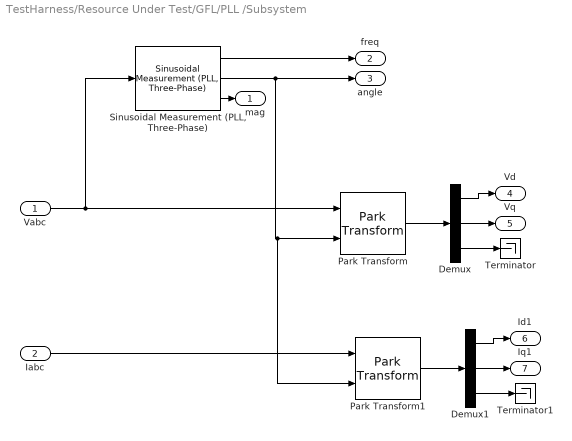
== system TestHarness/Resource Under Test/GFL/PLL /Subsystem ==
  Vabc : Inport
  Iabc : Inport  Port=2
  Demux : Demux  Outputs=3
  Demux1 : Demux  Outputs=3
  Park Transform : eeTransforms/Park Transform  AxisAlignment=Q-axis  PowerInvariant=on
  Park Transform1 : eeTransforms/Park Transform  AxisAlignment=Q-axis  PowerInvariant=on
  "Sinusoidal Measurement (PLL, Three-Phase)" : eeSinusoidalMeasurementV2/Sinusoidal Measurement (PLL, Three-Phase)  InputFilter=on  InputNormalization=off  Kp_LF=0.01  Ki_LF=2.05  F0=grid.frequency  Theta0=0  Ts=Ts
  Terminator : Terminator
  Terminator1 : Terminator
  mag : Outport
  freq : Outport  Port=2
  angle : Outport  Port=3
  Vd : Outport  Port=4
  Vq : Outport  Port=5
  Id1 : Outport  Port=6
  Iq1 : Outport  Port=7
  wires:
  Demux/3 -> Terminator/1
  Park Transform/1 -> Demux/1
  Demux/1 -> Vd/1
  Demux/2 -> Vq/1
  "Sinusoidal Measurement (PLL, Three-Phase)"/2 -> angle/1, Park Transform1/2, Park Transform/2
  "Sinusoidal Measurement (PLL, Three-Phase)"/1 -> freq/1
  "Sinusoidal Measurement (PLL, Three-Phase)"/3 -> mag/1
  Park Transform1/1 -> Demux1/1
  Demux1/1 -> Id1/1
  Demux1/2 -> Iq1/1
  Demux1/3 -> Terminator1/1
  Iabc/1 -> Park Transform1/1
  Vabc/1 -> "Sinusoidal Measurement (PLL, Three-Phase)"/1, Park Transform/1

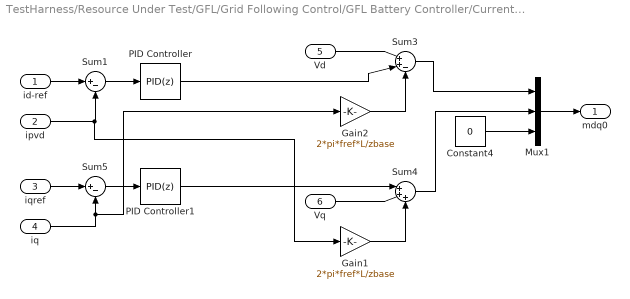
== system TestHarness/Resource Under Test/GFL/Grid Following Control/GFL Battery Controller/Current_controller ==
  id-ref : Inport
  ipvd : Inport  Port=2
  iqref : Inport  Port=3
  iq : Inport  Port=4
  Vd : Inport  Port=5
  Vq : Inport  Port=6
  Constant4 : Constant  Value=0
  Gain1 : Gain  Gain=2*pi*fref*L/zbase
  Gain2 : Gain  Gain=2*pi*fref*L/zbase
  Mux1 : Mux  Inputs=3
  PID Controller : slpidlib/PID Controller  Controller=PID  Form=Parallel  TimeDomain=Discrete-time  UseExternalTs=off  SampleTime=-1  IntegratorMethod=Forward Euler  FilterMethod=Forward Euler  ControllerParametersSource=internal  P=Kpic  I=Kiic  UseKiTs=off  D=Kd  UseExternalDerivativeSource=off  N=100  UseFilter=on  TunerSelectOption=Transfer Function Based (PID Tuner App)  InitialConditionSource=internal  InitialConditionForIntegrator=0  InitialConditionForFilter=0  DifferentiatorICPrevScaledInput=0  ExternalReset=none  TrackingMode=off  Kt=1  LimitOutput=off  SatLimitsSource=internal  UpperSaturationLimit=inf  LowerSaturationLimit=-inf  LinearizeAsGain=on  AntiWindupMode=none  Kb=1  LimitIntegrator=off  UpperIntegratorSaturationLimit=inf  LowerIntegratorSaturationLimit=-inf  POutMin=[]  POutMax=[]  IOutMin=[]  IOutMax=[]  DOutMin=[]  DOutMax=[]  NOutMin=[]  NOutMax=[]  SumOutMin=[]  SumOutMax=[]  SaturationOutMin=[]  SaturationOutMax=[]  PParamMin=[]  PParamMax=[]  IParamMin=[]  IParamMax=[]  DParamMin=[]  DParamMax=[]  NParamMin=[]  NParamMax=[]  KbParamMin=[]  KbParamMax=[]  KtParamMin=[]  KtParamMax=[]  KbOutMin=[]  KbOutMax=[]  KtOutMin=[]  KtOutMax=[]  IntegratorOutMin=[]  IntegratorOutMax=[]  FilterOutMin=[]  FilterOutMax=[]  SumI1OutMin=[]  SumI1OutMax=[]  SumI2OutMin=[]  SumI2OutMax=[]  SumI3OutMin=[]  SumI3OutMax=[]  SumI4OutMin=[]  SumI4OutMax=[]  SumDOutMin=[]  SumDOutMax=[]  DifferentiatorOutMin=[]  DifferentiatorOutMax=[]  FilterDiffOutCoefMin=[]  FilterDiffOutCoefMax=[]  ReciprocalOutMin=[]  ReciprocalOutMax=[]  SumDenOutMin=[]  SumDenOutMax=[]  SumNumOutMin=[]  SumNumOutMax=[]  DivideOutMin=[]  DivideOutMax=[]  UdiffTsProdOutMin=[]  UdiffTsProdOutMax=[]  NTsProdOutMin=[]  NTsProdOutMax=[]  UintegralTsProdOutMin=[]  UintegralTsProdOutMax=[]  UngainTsProdOutMin=[]  UngainTsProdOutMax=[]  ClampingZeroOutDataTypeStr=Inherit: Inherit via back propagation  ClampingZeroOutMin=[]  ClampingZeroOutMax=[]  FilterDenConstantOutDataTypeStr=Inherit: Inherit via back propagation  FilterDenConstantOutMin=[]  FilterDenConstantOutMax=[]  PCopyOutDataTypeStr=Inherit: Inherit via back propagation  PCopyOutMin=[]  PCopyOutMax=[]  NCopyOutDataTypeStr=Inherit: Inherit via back propagation  NCopyOutMin=[]  NCopyOutMax=[]  IntegratorContinuousStateAttributes=''  IntegratorStateMustResolveToSignalObject=off  IntegratorRTWStateStorageClass=Auto  FilterContinuousStateAttributes=''  FilterStateMustResolveToSignalObject=off  FilterRTWStateStorageClass=Auto  ParallelPVariant=InternalParameters  IdealPVariant=Disabled  IVariant=InternalParameters  DVariant=InternalParameters  IntegratorVariant=Discrete  SatVariant=Disabled  AWVariant=Passthrough  PCopyVariant=Disabled  TRVariant=Disabled  FdbkBlocksVariant=Forward  IdealPFdbkVariant=Disabled  SatFdbkVariant=Disabled  DerivativeFilterVariant=ForwardEulerFilter  NVariant=InternalParameters  NCopyVariant=Disabled  FilterICVariant=InternalICsFilter  IntegratorICVariant=InternalICs  ExternalResetVariant=Disabled  TRSumVariant=Passthrough  SumFdbkVariant=Disabled  SumVariant=Sum_PID  TsampFilterVariant=InternalTs  TsampNgainVariant=Passthrough  TsampIntegralVariant=Disabled_SignalSpec  ExternalSaturationOutDataTypeStr=Inherit: Same as second input  DerivativeSourceVariant=ErrorSignal  PreIntVariant=InternalPreInt
  PID Controller1 : slpidlib/PID Controller  Controller=PID  Form=Parallel  TimeDomain=Discrete-time  UseExternalTs=off  SampleTime=-1  IntegratorMethod=Forward Euler  FilterMethod=Forward Euler  ControllerParametersSource=internal  P=Kpic  I=Kiic  UseKiTs=off  D=Kd  UseExternalDerivativeSource=off  N=100  UseFilter=on  TunerSelectOption=Transfer Function Based (PID Tuner App)  InitialConditionSource=internal  InitialConditionForIntegrator=0  InitialConditionForFilter=0  DifferentiatorICPrevScaledInput=0  ExternalReset=none  TrackingMode=off  Kt=1  LimitOutput=off  SatLimitsSource=internal  UpperSaturationLimit=inf  LowerSaturationLimit=-inf  LinearizeAsGain=on  AntiWindupMode=none  Kb=1  LimitIntegrator=off  UpperIntegratorSaturationLimit=inf  LowerIntegratorSaturationLimit=-inf  POutMin=[]  POutMax=[]  IOutMin=[]  IOutMax=[]  DOutMin=[]  DOutMax=[]  NOutMin=[]  NOutMax=[]  SumOutMin=[]  SumOutMax=[]  SaturationOutMin=[]  SaturationOutMax=[]  PParamMin=[]  PParamMax=[]  IParamMin=[]  IParamMax=[]  DParamMin=[]  DParamMax=[]  NParamMin=[]  NParamMax=[]  KbParamMin=[]  KbParamMax=[]  KtParamMin=[]  KtParamMax=[]  KbOutMin=[]  KbOutMax=[]  KtOutMin=[]  KtOutMax=[]  IntegratorOutMin=[]  IntegratorOutMax=[]  FilterOutMin=[]  FilterOutMax=[]  SumI1OutMin=[]  SumI1OutMax=[]  SumI2OutMin=[]  SumI2OutMax=[]  SumI3OutMin=[]  SumI3OutMax=[]  SumI4OutMin=[]  SumI4OutMax=[]  SumDOutMin=[]  SumDOutMax=[]  DifferentiatorOutMin=[]  DifferentiatorOutMax=[]  FilterDiffOutCoefMin=[]  FilterDiffOutCoefMax=[]  ReciprocalOutMin=[]  ReciprocalOutMax=[]  SumDenOutMin=[]  SumDenOutMax=[]  SumNumOutMin=[]  SumNumOutMax=[]  DivideOutMin=[]  DivideOutMax=[]  UdiffTsProdOutMin=[]  UdiffTsProdOutMax=[]  NTsProdOutMin=[]  NTsProdOutMax=[]  UintegralTsProdOutMin=[]  UintegralTsProdOutMax=[]  UngainTsProdOutMin=[]  UngainTsProdOutMax=[]  ClampingZeroOutDataTypeStr=Inherit: Inherit via back propagation  ClampingZeroOutMin=[]  ClampingZeroOutMax=[]  FilterDenConstantOutDataTypeStr=Inherit: Inherit via back propagation  FilterDenConstantOutMin=[]  FilterDenConstantOutMax=[]  PCopyOutDataTypeStr=Inherit: Inherit via back propagation  PCopyOutMin=[]  PCopyOutMax=[]  NCopyOutDataTypeStr=Inherit: Inherit via back propagation  NCopyOutMin=[]  NCopyOutMax=[]  IntegratorContinuousStateAttributes=''  IntegratorStateMustResolveToSignalObject=off  IntegratorRTWStateStorageClass=Auto  FilterContinuousStateAttributes=''  FilterStateMustResolveToSignalObject=off  FilterRTWStateStorageClass=Auto  ParallelPVariant=InternalParameters  IdealPVariant=Disabled  IVariant=InternalParameters  DVariant=InternalParameters  IntegratorVariant=Discrete  SatVariant=Disabled  AWVariant=Passthrough  PCopyVariant=Disabled  TRVariant=Disabled  FdbkBlocksVariant=Forward  IdealPFdbkVariant=Disabled  SatFdbkVariant=Disabled  DerivativeFilterVariant=ForwardEulerFilter  NVariant=InternalParameters  NCopyVariant=Disabled  FilterICVariant=InternalICsFilter  IntegratorICVariant=InternalICs  ExternalResetVariant=Disabled  TRSumVariant=Passthrough  SumFdbkVariant=Disabled  SumVariant=Sum_PID  TsampFilterVariant=InternalTs  TsampNgainVariant=Passthrough  TsampIntegralVariant=Disabled_SignalSpec  ExternalSaturationOutDataTypeStr=Inherit: Same as second input  DerivativeSourceVariant=ErrorSignal  PreIntVariant=InternalPreInt
  Sum1 : Sum  Inputs=|+-
  Sum3 : Sum  Inputs=|++-
  Sum4 : Sum  Inputs=|+++
  Sum5 : Sum  Inputs=|+-
  mdq0 : Outport
  wires:
  PID Controller/1 -> Sum3/2
  Sum3/1 -> Mux1/1
  Gain2/1 -> Sum3/3
  ipvd/1 -> Gain1/1, Sum1/2
  id-ref/1 -> Sum1/1
  Gain1/1 -> Sum4/3
  Vq/1 -> Sum4/2
  iq/1 -> Gain2/1, Sum5/2
  Sum1/1 -> PID Controller/1
  Vd/1 -> Sum3/1
  Constant4/1 -> Mux1/3
  Sum5/1 -> PID Controller1/1
  iqref/1 -> Sum5/1
  PID Controller1/1 -> Sum4/1
  Sum4/1 -> Mux1/2
  Mux1/1 -> mdq0/1
